simulink model "SDR_Model"  (R2022a)
settings: Solver=VariableStepAuto  StartTime=0.0  StopTime=10  RelTol=1e-3
model workspace (MAT data in the model file):
  fs = 10000
undefined symbols (not defined in the file): daq
libraries: daqlib x3, dspsnks4 x1, dspstat3 x1
settings Model: Creator=FIT UBD  LastModifiedBy=FIT UBD

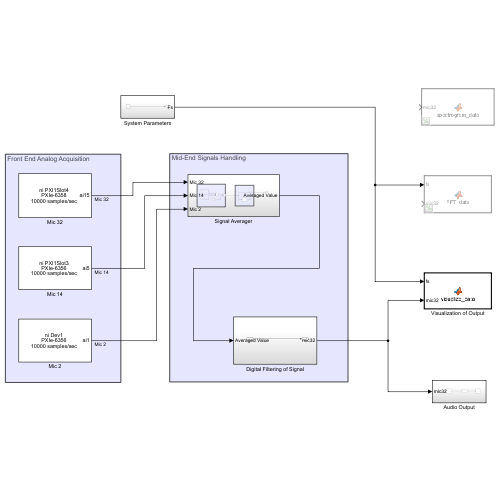
[thumbnail: Simulink's stored preview of the top-level diagram]
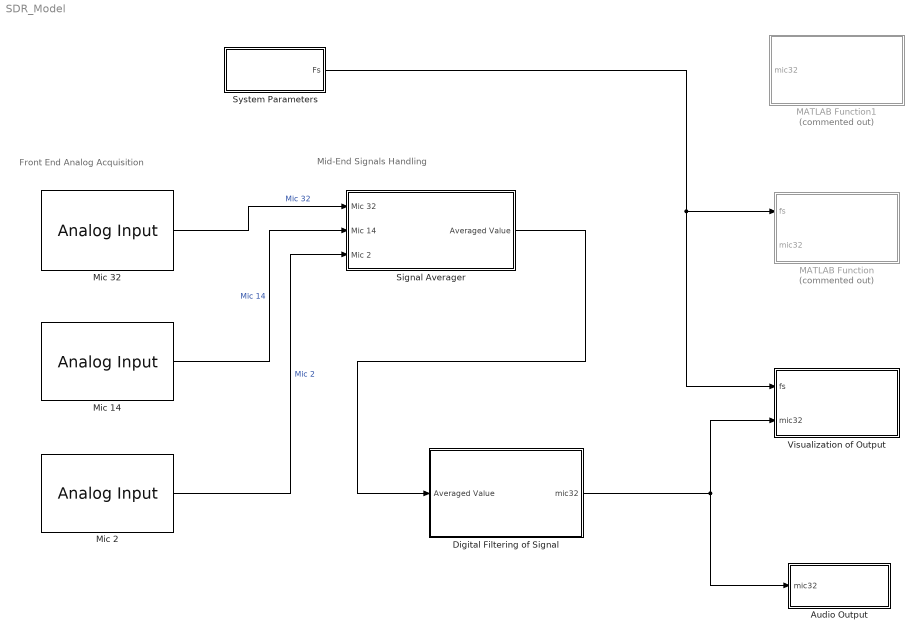
== system SDR_Model ==
  note: Mid-End Signals Handling
  note: Front End Analog Acquisition
  Audio Output : Subsystem
  Digital Filtering of Signal : Subsystem
  MATLAB Function : MATLAB Function  Commented=on  TreatAsAtomicUnit=on
  MATLAB Function1 : MATLAB Function  Commented=on  TreatAsAtomicUnit=on
  Mic 14 : daqlib/Analog Input  DeviceMenu=(none)  Device=ni PXI1Slot3 (PXIe-6356)  ObjConstructor=daq.createSession('ni')  NChannelsSelected=1  Channels=0$ai0$$PXI1Slot3$1$4$1$1$#0$ai1$$PXI1Slot3$1$4$1$1$#0$ai2$$PXI1Slot3$1$4$1$1$#0$ai3$$PXI1Slot3$1$4$1$1$#0$ai4$$PXI1Slot3$1$4$1$1$#1$ai5$$PXI1Slot3$1$4$1$1$#0$ai6$$PXI1Slot3$1$4$1$1$#0$ai7$$PXI1Slot3$1$4$1$1$#  NPorts=1 per channel  SampleRate=10000  ActualRate=10000  ScansPerTrigger=600  OutputTimestamp=off  AcqMode=1  NumFrameBuffer=100  OutputTriggertime=off
      settings: SourceProductBaseCode=DA
  Mic 2 : daqlib/Analog Input  DeviceMenu=(none)  Device=ni Dev1 (PXIe-6356)  ObjConstructor=daq.createSession('ni')  NChannelsSelected=1  Channels=0$ai0$$Dev1$1$4$1$1$#1$ai1$$Dev1$1$4$1$1$#0$ai2$$Dev1$1$4$1$1$#0$ai3$$Dev1$1$4$1$1$#0$ai4$$Dev1$1$4$1$1$#0$ai5$$Dev1$1$4$1$1$#0$ai6$$Dev1$1$4$1$1$#0$ai7$$Dev1$1$4$1$1$#  NPorts=1 per channel  SampleRate=10000  ActualRate=10000  ScansPerTrigger=600  OutputTimestamp=off  AcqMode=0  NumFrameBuffer=100  OutputTriggertime=off
      settings: SourceProductBaseCode=DA
  Mic 32 : daqlib/Analog Input  DeviceMenu=(none)  Device=ni PXI1Slot4 (PXIe-6358)  ObjConstructor=daq.createSession('ni')  NChannelsSelected=1  Channels=0$ai0$$PXI1Slot4$1$4$1$1$#0$ai1$$PXI1Slot4$1$4$1$1$#0$ai2$$PXI1Slot4$1$4$1$1$#0$ai3$$PXI1Slot4$1$4$1$1$#0$ai4$$PXI1Slot4$1$4$1$1$#0$ai5$$PXI1Slot4$1$4$1$1$#0$ai6$$PXI1Slot4$1$4$1$1$#0$ai7$$PXI1Slot4$1$4$1$1$#0$ai8$$PXI1Slot4$1$4$1$1$#0$ai9$$PXI1Slot4$1$4$1$1$#0$ai10$$PXI1Slot4$1$4$1$1$#0$ai11$$PXI1Slot4$1$4$1$1$#0$ai12$$PXI1Slot4$1$4$1$1$#0$ai13$$PXI1Slot4$1$4$1$1$#0$ai14$$PXI1Slot4$1$4$1$1$#1$ai15$$PXI1Slot4$1$4$1$1$#  NPorts=1 per channel  SampleRate=10000  ActualRate=10000  ScansPerTrigger=600  OutputTimestamp=off  AcqMode=1  NumFrameBuffer=100  OutputTriggertime=off
      settings: SourceProductBaseCode=DA
  Signal Averager : Subsystem
  System Parameters : Subsystem
  Visualization of Output : MATLAB Function  TreatAsAtomicUnit=on
  wires:
  System Parameters/1(Fs) -> Visualization of Output/1(fs), MATLAB Function/1(fs)
  Mic 2/1 -> Signal Averager/3(Mic 2)  "Mic 2"
  Mic 32/1 -> Signal Averager/1(Mic 32)  "Mic 32"
  Mic 14/1 -> Signal Averager/2(Mic 14)  "Mic 14"
  Signal Averager/1(Averaged Value) -> Digital Filtering of Signal/1(Averaged Value)
  Digital Filtering of Signal/1(mic32) -> Audio Output/1(mic32), Visualization of Output/2(mic32)

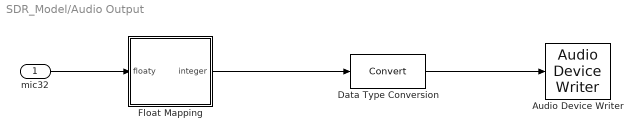
== system SDR_Model/Audio Output ==
  mic32 : Inport
  Audio Device Writer : dspsnks4/Audio Device Writer  Driver=DirectSound  Device=Default  InheritSampleRate=on  SampleRate=44100  BitDepth=16-bit integer  BufferSize=4096  NumBuffers=10  DefaultOutputChannelMapping=on  OutputChannelMapping=1:2  OutputNumUnderrunSamples=off  DriverIdx=1  DeviceWarnFlag=''
  Data Type Conversion : DataTypeConversion  SaturateOnIntegerOverflow=off  RndMeth=Floor
  Float Mapping : MATLAB Function  TreatAsAtomicUnit=on
  wires:
  mic32/1 -> Float Mapping/1(floaty)
  Float Mapping/1(integer) -> Data Type Conversion/1
  Data Type Conversion/1 -> Audio Device Writer/1

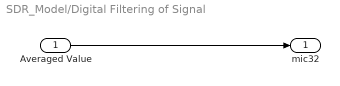
== system SDR_Model/Digital Filtering of Signal ==
  Averaged Value : Inport
  mic32 : Outport
  wires:
  Averaged Value/1 -> mic32/1

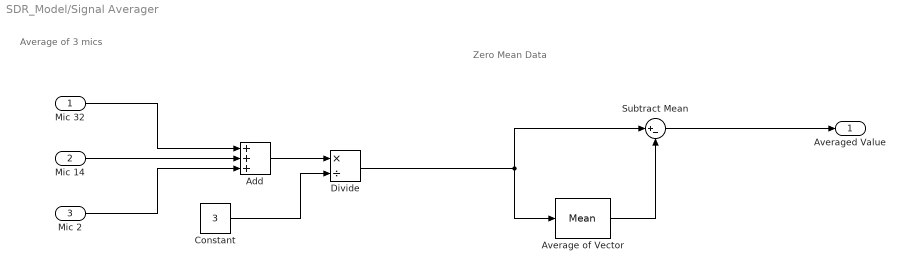
== system SDR_Model/Signal Averager ==
  note: Zero Mean Data
  note: Average of 3 mics
  Mic 32 : Inport
  Mic 14 : Inport  Port=2
  Mic 2 : Inport  Port=3
  Add : Sum  Inputs=+++
  Average of Vector : dspstat3/Mean  run=off  InputProcessing=Columns as channels (frame based)  reset_popup=None  directionMode=Each column  dimension=1  roiEnable=off  roiType=Rectangles  roiPortion=Entire ROI  roiOutput=Individual statistics for each ROI  roiFlag=off  roundingMode=Floor  overflowMode=off  outputDataTypeStr=Inherit: Same as accumulator  outputMin=[]  outputMax=[]  outputLastDataTypeStr=Inherit: Same as accumulator
  Constant : Constant  Value=3
  Divide : Product  Inputs=*/
  Subtract Mean : Sum  Inputs=|+-
  Averaged Value : Outport
  wires:
  Mic 32/1 -> Add/1
  Mic 14/1 -> Add/2
  Mic 2/1 -> Add/3
  Add/1 -> Divide/1
  Constant/1 -> Divide/2
  Divide/1 -> Subtract Mean/1, Average of Vector/1
  Average of Vector/1 -> Subtract Mean/2
  Subtract Mean/1 -> Averaged Value/1

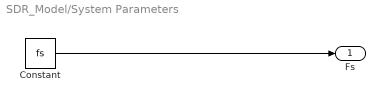
== system SDR_Model/System Parameters ==
  Constant : Constant  Value=fs
  Fs : Outport
  wires:
  Constant/1 -> Fs/1

== matlab function SDR_Model/Visualization of Output ==
  data: fs input; mic32 input
function visualize_data(fs, mic32)
 
% --Data memory for the SDR
    persistent data

    if isempty(data)
        data = [];
    end

% --Save data for maximum time length
    data = [mic32; data];

% --Define x values
    time = (1/fs)*(0:length(data) - 1);
        
% --Plot data
    figure(1)
    plot(time, data)
        xlim([0 0.5])
        ylim([-0.1 0.1])
        grid on
        xlabel("Time (s)")
        title("Time history of Waveform")

% --Reformat data length
    if length(data) >= 0.5*fs - length(mic32)
        data = data(1:0.5*fs - length(mic32));
    end

end

== matlab function SDR_Model/MATLAB Function1 ==
  data: mic32 input
function spectrogram_data(mic32)

end

== matlab function SDR_Model/Audio Output/Float Mapping ==
  data: floaty input; integer output
function integer = float_map(floaty)

% --Round all values

% --Convert to integers
    b = floaty .* 1000;

% --Round to whole int
    integer = round(b);

end

== matlab function SDR_Model/MATLAB Function ==
  data: fs input; mic32 input
function FFT_data(fs, mic32)

% --Initialize
    persistent i ff frequency

% --Take FFT of data
    f_data_mag = [abs(fft(mic32))]';
    f_data_amp = 2*f_data_mag/length(f_data_mag);
        
% --Plot data
    if isempty(i)
        % --Define Freq
            N = length(f_data_amp);
            T = N/fs;
            frequency = (1/T)*(0:N-1);

        % --Plot
            figure(2)
            ff = plot(frequency, f_data_amp);
                xlim([0 fs/2])
                xlabel('Frequency (Hz)')
                ylabel('Amplitude')
                grid on
                title('Real Time Frequency Spectra')
                ylim([0 0.05])

        % --Update
        i = [1 1];
    end

% --Link
    ff.XDataSource = 'frequency';
    ff.YDataSource = 'f_data_amp';

% --Update
    refreshdata

end
